simulink model "IEEE34bus_2subsystem"  (R2022b)
settings: Solver=ode4  StartTime=0.0  StopTime=inf  FixedStep=Ts  MaxStep=1e-4  RelTol=1e-4
InitFcn:
  | a=1; % Loading Factor
  | Ts=50e-6;
  | % phase to sequence conversion of RXB matrices
  | c=1*exp(sqrt(-1)*(120*pi/180));
  | T=[1 1 1;1 c*c c;1 c c*c];
  | Tinv=1/3*[1 1 1;1 c c*c;1 c*c c];
  | 
  | % Simulation data for the IEEE 34 Node Test Feeder model
  | mi2km = 1.60934;%  miles to km conversion
  | ft2km = 0.0003048; % feet to km conversion
  | ms2F = 1*1e-6/(2*pi*60);% microsiemens to Farads conversion
  | 
  | %% Configuration 300 - series reactance - ohm/mile
  | R_300 = [1.3368 0.2101 0.2130;0.2101 1.3238 0.2066;0.2130 0.2066 1.3294];
  | X_300 = [1.3343 0.5779 0.5015;0.5779 1.3569 0.4591;0.5015 0.4591 1.3471];
  | % charging susceptance - microsiemens/mile
  | B_300 = [5.3350 -1.5313 -0.9943;-1.5313 5.0979 -0.6212;-0.9943 -0.6212 4.8880];
  | 
  | R_300 = R_300/mi2km;
  | Rseq=Tinv*R_300*T;
  | R1_300=Rseq(2,2);R0_300=Rseq(1,1);
  | 
  | L_300 = (X_300/(2*pi*60))/mi2km;
  | Lseq=Tinv*L_300*T;
  | L1_300=Lseq(2,2);L0_300=Lseq(1,1);
  | 
  | C_300 =(B_300*ms2F)/mi2km;
  | Cseq=Tinv*C_300*T;
  | C1_300=Cseq(2,2);C0_300=Cseq(1,1);
  | 
  | %% Configuration 301 - series reactance - ohm/mile
  | R_301 = [1.9300 0.2327 0.2359;0.2327 1.9157 0.2288;0.2359 0.2288 1.9219];
  | X_301 = [1.4115 0.6442 0.5691;0.6442 1.4281 0.5238;0.5691 0.5238 1.4209];
  | % charging susceptance - microsiemens/mile
  | B_301 = [5.1207 -1.4364 -0.9402;-1.4364 4.9055 -0.5951;-0.9402 -0.5951 4.7154];
  | 
  | R_301 = R_301/mi2km;
  | Rseq=Tinv*R_301*T;
  | R1_301=Rseq(2,2);R0_301=Rseq(1,1);
  | 
  | L_301 = (X_301/(2*pi*60))/mi2km;
  | Lseq=Tinv*L_301*T;
  | L1_301=Lseq(2,2);L0_301=Lseq(1,1);
  | 
  | C_301 =(B_301*ms2F)/mi2km;
  | Cseq=Tinv*C_301*T;
  | C1_301=Cseq(2,2);C0_301=Cseq(1,1);
  | 
  | %% Configuration 302 - series reactance - ohm/mile
  | R_302 = [2.7995 0 0;0 0 0;0 0 0];
  | X_302 = [1.4855 0 0;0 0 0;0 0 0];
  | % charging susceptance - microsiemens/mile
  | B_302 = [4.2251 0 0;0 0 0;0 0 0];
  | 
  | R_302 = R_302/mi2km;
  | Rseq=Tinv*R_302*T;
  | R1_302=Rseq(2,2);R0_302=Rseq(1,1);
  | 
  | L_302 = (X_302/(2*pi*60))/mi2km;
  | Lseq=Tinv*L_302*T;
  | ... (+41 lines)
undefined symbols (not defined in the file): find_system, I, Left, MOV_segment19, MOV_segment9, powergui, Right, type, V, X, xn_g1
libraries: spsSeriesRLCBranchLib x75, spsGroundLib x70, spsThreePhaseVIMeasurementLib x37, spsVoltageMeasurementLib x36, spsThreePhaseSeriesRLCLoadLib x32, spsThreePhasePISectionLineLib x24, spsDCVoltageSourceLib x24, ssn_lib x16, spsSeriesRLCLoadLib x14, spsACCurrentSourceLib x12, spsOnDelayLib x12, spsPiSectionLineLib x8
(part 4 of 8)

== system IEEE34bus_2subsystem/SM_34p/Regulator 3/Single Phase SVR_A/Transformer with Taps ==
  note: Vsec on Pt Ratio base
  note: Isec on CT Ratio base
  N : Inport
  "   " : Terminator
  "    " : Gain  Gain=1/ptRatio
  " 1" : Gain  Gain=-1/ctRatio
  Back-Euler : Constant
  CT1 : spsCurrentMeasurementLib/Current Measurement  PhasorSimulation=off  OutputType=Complex  PSBequivalent=0
  Fcn : Fcn  Expr=1+0.1*u(1)/16
  Ground1 : spsGroundLib/Ground  LConnTagsString=a
  Memory : Memory
  Memory1 : Memory
  Mux1 : Mux  Inputs=2
  PT : spsVoltageMeasurementLib/Voltage Measurement  PhasorSimulation=off  OutputType=Complex  PSBequivalent=0
  SSN Interface Block (1ph) : ssn_lib/SSN Interface Block (1ph)  nb_phase=1  nb_port=2  p1_type=I-type(Left)  p2_type=X-type(Right)  p3_type=V-type(Left)  p4_type=V-type(Left)  p5_type=V-type(Left)  p6_type=V-type(Left)  p7_type=V-type(Left)  p8_type=V-type(Left)  p9_type=V-type(Left)  p10_type=V-type(Left)  p11_type=V-type(Left)  p12_type=V-type(Left)  p13_type=V-type(Left)  p14_type=V-type(Left)  p15_type=V-type(Left)  p16_type=V-type(Left)  I_port_shunt_resistance=1e9
  SSN Interface Block (1ph)2 : ssn_lib/SSN Interface Block (1ph)  nb_phase=1  nb_port=2  p1_type=X-type(Left)  p2_type=I-type(Right)  p3_type=X-type(Left)  p4_type=V-type (Right)  p5_type=V-type(Left)  p6_type=V-type(Left)  p7_type=V-type(Left)  p8_type=V-type(Left)  p9_type=V-type(Left)  p10_type=V-type(Left)  p11_type=V-type(Left)  p12_type=V-type(Left)  p13_type=V-type(Left)  p14_type=V-type(Left)  p15_type=V-type(Left)  p16_type=V-type(Left)  I_port_shunt_resistance=1e9
  SSN OLTC xfo v2 : Subsystem  AncestorBlock=artemis/SSN/SSN OLTC/SSN OLTC xfo v2  mask(Norton-Type External Nodal Subsystem){nnode=2, taggg=ce4x9218xa137594c517a, conntype=2 ports, RLpri=[1e-3 1e-4], Rcore=10000, ensat=off, Lcore=100, Lsat=1, phisat=100, Ts=Ts}
      mask prompts: nnode "Number of Electric nodes"; taggg "Unique Tag Identifier (automatic)"; conntype "Connection type"; RLpri "Primary winding resistance and inductance ([Ohms H])"; Rcore "Core Resistance (Ohms)"; ensat "Enable Saturation"; Lcore "Unsaturated magnetisation inductance (H)"; Lsat "Saturated magnetisation inductance (H)"; phisat "Flux saturation threshold (Weber)"; Ts "Sample Time (s)"
      mask help:
      | Continuously-variable On-Load Tapped Transformer (OLTC) (SSN Custom model)
      |
      | This block implements a 2 winding OLTC saturable transformer in SSN.
      | The model has a variable secondary inductance and resistance as well as turn-ratio.
      | The secondary winding is on the side marked with 'TAP'
      |
      | Mask parameters:
      |    Unique Tag Identifier: unique tag required by SSN to recknonize SSN external models
      |    Primary winding resistance and inductance ([Ohms H])
      |    Core Resistance (Ohms)
      |    Unsaturated magnetisation inductance (H): unsaturated core magnetization inductance
      |    Saturated magnetisation inductance (H): local inductance of the core in the saturated region
      |    Flux saturation threshold (Weber): flux saturation point
      |
      | Signal parameters:
      |
      | Signal inputs:
      |    1st sig: secondary winding resistance (Ohms)
      |    2nd sig: secondary winding inductance (H)
      |    3rd sig: transformer turn ratio k (V_secondary_tapped=k*V_primary)
      |    4th sig:  when set to 1, uses the Backward Euler method for solver. This can be used dynamically during simulation for example to damp numerical oscillations after switching events or after tap changes.
      |
      | Signals ouputs:
      |    1st signal: primary input current (A)
      |    2nd signal: secondary winding current (A)
      |    3rd signal: transformer flux (Wb)
      |
      | Saturation characteristic:
      |          flux
      |             ^              2
      |             |      1       *   <--- slope between point1 and point2 is Lsaturated
      |  phisat  |-----*  <---  this is the knee of flux=f(imag)
      |             |
      |             |
      |             |  <-----slope between origin and point1 is Lunsaturated
      |             *-------------------> imag
      mask init:
      | bloc=gcb;
      | taggg=get_param(bloc,'taggg');
      | conntyp=get_param(bloc,'conntype');
      | set_param([bloc '/FromV'],'GotoTag',['ssn_ext_sys_from_V_' taggg]);
      | set_param([bloc '/GotoHist'],'GotoTag',['ssn_ext_sys_goto_Hist_' taggg]);
      | set_param([bloc '/GotoY'],'GotoTag',['ssn_ext_sys_goto_Y_' taggg]);
      | 
      | R1=RLpri(1);
      | L1=RLpri(2);
      | 
      | if isequal(get_param(bloc,'ensat'),'off')
      |     phisat=1e20;
      | end
      | 
      | if isequal(conntyp,'4 ports')
      |     vin_sel=[1 2 3 4];
      |     Vinzeros=0;
      |     hist_sel=[1 2 3 4];
      |     a1=0;a2=0;a3=100;a4=100; b1=[7,34,40,33,31,33,40,33,31,33,40,33,31,33,40,34,7];b2=[30,30,34,42,40,37,45,52,50,47,54,62,59,57,65,70,70];b3=[93,67,60,67,70,67,60,67,70,67,60,67,70,67,60,67,93];b4=[30,30,34,42,40,37,45,52,50,47,54,62,60,57,65,70,70];
      |     c1=[20,20]*0;c2=[20,30]*0;c3=[27,14]*0;c4=[20,20]*0;c5=[24,17]*0;c6=[16,16]*0;c7=[22,19]*0;c8=[13,13]*0;c9=[80,80]*0;c10=[20,30]*0;c11=[88,74]*0;c12=[20,20]*0;c13=[85,77]*0;c14=[16,16]*0;c15=[81,79]*0;c16=[13,13]*0;
      |     %d1=[85,80];d2=[60,60];d3=[83,83];d4=[50,60];d5=[90,88,86];d6=[50,60,50];d7=[89,87];d8=[54,54];d9=[92,95,96,96,95,92,92];d10=[53,53,55,58,60,60,50];
      | 
      | 
      | elseif isequal(conntyp,'3 ports (primary grounded)')
      |     vin_sel=[1 2 5 3];
      |     Vinzeros=[0 0];
      |     hist_sel=[1 2 4];
      |   
      |      a1=0;a2=0;a3=100;a4=100; b1=[20,34,40,33,31,33,40,33,31,33,40,33,31,33,40,34,7];b2=[30,30,34,42,40,37,45,52,50,47,54,62,59,57,65,70,70];b3=[93,67,60,67,70,67,60,67,70,67,60,67,70,67,60,67,93];b4=[30,30,34,42,40,37,45,52,50,47,54,62,60,57,65,70,70];
      |     c1=[20,20];c2=[20,30];c3=[27,14];c4=[20,20];c5=[24,17];c6=[16,16];c7=[22,19];c8=[13,13];c9=[80,80]*0;c10=[20,30]*0;c11=[88,74]*0;c12=[20,20]*0;c13=[85,77]*0;c14=[16,16]*0;c15=[81,79]*0;c16=[13,13]*0;
      |     %d1=[85,80];d2=[60,60];d3=[83,83];d4=[50,60];d5=[90,88,86];d6=[50,60,50];d7=[89,87];d8=[54,54];d9=[92,95,96,96,95,92,92];d10=[53,53,55,58,60,60,50];
      | elseif isequal(conntyp,'3 ports (tapped secondary grounded)')
      |     vin_sel=[1 2 3 5];
      |     Vinzeros=[0 0];
      |     hist_sel=[1 2 3];
      |  
      |    a1=0;a2=0;a3=100;a4=100; b1=[20,34,40,33,31,33,40,33,31,33,40,33,31,33,40,34,7];b2=[30,30,34,42,40,37,45,52,50,47,54,62,59,57,65,70,70];b3=[80,67,60,67,70,67,60,67,70,67,60,67,70,67,60,67,93];b4=[30,30,34,42,40,37,45,52,50,47,54,62,60,57,65,70,70];
      |     c1=[20,20]*0;c2=[20,30]*0;c3=[27,14]*0;c4=[20,20]*0;c5=[24,17]*0;c6=[16,16]*0;c7=[22,19]*0;c8=[13,13]*0;c9=[80,80];c10=[20,30];c11=[88,74];c12=[20,20];c13=[85,77];c14=[16,16];c15=[81,79];c16=[13,13];
      |     %d1=[85,80];d2=[60,60];d3=[83,83];d4=[50,60];d5=[90,88,86];d6=[50,60,50];d7=[89,87];d8=[54,54];d9=[92,95,96,96,95,92,92];d10=[53,53,55,58,60,60,50];
      | elseif isequal(conntyp,'2 ports')
      |     vin_sel=[1 2 5 5];
      |     Vinzeros=[0 0 0];
      |     hist_sel=[1 2];
      |         a1=0;a2=0;a3=100;a4=100; b1=[20,34,40,33,31,33,40,33,31,33,40,33,31,33,40,34,7];b2=[30,30,34,42,40,37,45,52,50,47,54,62,59,57,65,70,70];b3=[80,67,60,67,70,67,60,67,70,67,60,67,70,67,60,67,93];b4=[30,30,34,42,40,37,45,52,50,47,54,62,60,57,65,70,70];
      |     c1=[20,20];c2=[20,30];c3=[27,14];c4=[20,20];c5=[24,17];c6=[16,16];c7=[22,19];c8=[13,13];c9=[80,80];c10=[20,30];c11=[88,74];c12=[20,20];c13=[85,77];c14=[16,16];c15=[81,79];c16=[13,13];
      |     %d1=[85,80];d2=[60,60];d3=[83,83];d4=[50,60];d5=[90,88,86];d6=[50,60,50];d7=[89,87];d8=[54,54];d9=[92,95,96,96,95,92,92];d10=[53,53,55,58,60,60,50];
      | else
      | 
      | end
      | 
      | ori=get_param(bloc,'Orientation');
      | 
      | if isequal(ori,'right')
      |     d1=[73,67];d2=[56,56];d3=[70,70];d4=[45,56];d5=[80,77,75];d6=[45,56,45];d7=[79,76];d8=[50,50];d9=[82,84,86,84,82,82];d10=[50,50,54,56,56,45];
      | else
      |     d1=[73,71,69,71,73,73];d2=[50,50,52,56,56,45];d3=[80,77,75];d4=[45,56,45];d5=[76,79];d6=[50,50];d7=[88,82];d8=[56,56];d9=[85,85];d10=[45,56];
      | end
      settings: LibrarySourceBlock=artemis/SSN/SSN OLTC/SSN OLTC xfo v2
      settings: CopyFcn=|
      | str=tempname;
      | str=strrep(str(end-20:end),'_','x');
      | set_param(gcb,'taggg',str);
      | set_param(gcb,'LinkStatus','inactive');
      mask Help: eval('open SSN_OLTC.pdf;');
      mask TypeOptions conntype: 4 ports | 3 ports (primary grounded) | 3 ports (tapped secondary grounded) | 2 ports
      mask Callback conntype:
      | bloc=gcb;
      | conntyp=get_param(bloc,'conntype');
      | nn=fts6_xfo_port_cb(bloc,conntyp);
      | set_param(bloc,'nnode',nn);
      mask Display:
      | plot(a1,a2,a3,a4,b1,b2,b3,b4,c1,c2,c3,c4,c5,c6,c7,c8,c9,c10,c11,c12,c13,c14,c15,c16);
      | color('blue');
      | plot(d1,d2,d3,d4,d5,d6,d7,d8,d9,d10);
  Transfo R2-L2-turnratio : Constant  Value=[0.0001 0.00001 1]
  x : Product  RndMeth=Zero
  L : PMIOPort  Tag=PMCPort  Side=Right
  S : PMIOPort  Port=2  Side=Left
  Isec : Outport
  Vsec : Outport  Port=2
  wires:
  Fcn/1 -> x/1
  Mux1/1 -> SSN OLTC xfo v2/1(params)
  x/1 -> Mux1/1
  Transfo R2-L2-turnratio/1 -> x/2
  Back-Euler/1 -> Mux1/2
  SSN OLTC xfo v2/1(meas) -> "   "/1  "transfo flux (Weber)"
  N/1 -> Fcn/1
  "    "/1 -> Memory1/1
  PT/1 -> "    "/1
  CT1/1 -> " 1"/1
  " 1"/1 -> Memory/1
  Memory1/1 -> Vsec/1
  Memory/1 -> Isec/1
  connections:
  CT1/RConn1 -- SSN Interface Block (1ph)2/RConn1 -- PT/LConn1
  SSN OLTC xfo v2/LConn1 -- SSN Interface Block (1ph)/RConn1
  SSN OLTC xfo v2/RConn1 -- SSN Interface Block (1ph)2/LConn1
  S/RConn1 -- SSN Interface Block (1ph)/LConn1
  PT/LConn2 -- Ground1/LConn1
  CT1/LConn1 -- L/RConn1

== system IEEE34bus_2subsystem/SM_34p/Regulator 3/Single Phase SVR_A/Voltage Regulator Control ==
  Vm : Inport
  Constant : Constant  Value=RegulatorOn
  Tap Changer Control : Subsystem  mask(Tap Changer Control){MinMaxTap=TapMinMax, InitialPosition=InitialTap, MecDelay=TapSelectionTime}
      mask prompts: MinMaxTap "Minimum and maximum tap number [ Min  Max ] :"; InitialPosition "Initial tap position"; MecDelay "Mechanical delay time"
      mask init:
      | if MecDelay<=0,
      | 	MecDelay=1/60;
      | end
  Voltage regulator : Subsystem  mask{Vref=RegulatorVref*120, DeadBand=RegulatorDeadBand*120, TimeDelay=RegulatorDelay}
      mask prompts: Vref "Vref (on 120v base)"; DeadBand "Deadband (on 120v base)"; TimeDelay "Time delay (s)"
  N : Outport
  Tap : Outport  Port=2
  wires:
  Voltage regulator/2(Down) -> Tap Changer Control/2("Down ")
  Tap Changer Control/1(TapNo) -> Tap/1, N/1  "Tap"
  Voltage regulator/1(Up) -> Tap Changer Control/1("Up ")
  Tap Changer Control/2(Ready) -> Voltage regulator/2(Ready)
  Constant/1 -> Voltage regulator/3(RegOn)
  Vm/1 -> Voltage regulator/1(Vmes (pu))

== system IEEE34bus_2subsystem/SM_34p/Regulator 3/Single Phase SVR_B/Line Drop Compensator ==
  note: Vm=Vsec-Isec(Rc+jXc)
  Isec : Inport
  Vsec : Inport  Port=2
  "        " : spsLinearTransformerLib/Linear Transformer  UNITS=SI  NominalPower=[pNom fNom]  winding1=[vNom/ptRatio 1e-7 1e-8]  winding2=[vNom/ptRatio 1e-7 1e-8]  ThreeWindings=off  winding3=[3.15e+005 0.7938 0.084225]  RmLm=[1e5 1e5]  Measurements=None  DataType=on
  "CTS  " : spsControlledCurrentSourceLib/Controlled Current Source  Initialize=on  Source_Type=AC  Amplitude=0  Phase=0  Frequency=0  Measurements=None
  "PTS  " : spsControlledVoltageSourceLib/Controlled Voltage Source  Initialize=on  Source_Type=AC  Amplitude=0  Phase=0  Frequency=0  Measurements=None
  RMS : spsRMSLib/RMS  TrueRMS=on  Freq=60  RMSInit=120  Ts=0
  Raux : spsSeriesRLCBranchLib/Series RLC Branch  LConnTagsString=__new0  RConnTagsString=__new0  BranchType=R  Resistance=1e3  Inductance=1.6 / (120*pi)  SetiL0=off  InitialCurrent=0  Capacitance=1e-6  Setx0=off  InitialVoltage=0  Measurements=None
  Rc+jXc : spsSeriesRLCBranchLib/Series RLC Branch  LConnTagsString=__new0  RConnTagsString=__new0  BranchType=RL  Resistance=Rc  Inductance=Xc / (2*pi*fNom)  SetiL0=off  InitialCurrent=0  Capacitance=1e-6  Setx0=off  InitialVoltage=0  Measurements=None
  VRelay : spsVoltageMeasurementLib/Voltage Measurement  PhasorSimulation=off  OutputType=Complex  PSBequivalent=0
  Vm : Outport
  wires:
  RMS/1 -> Vm/1
  VRelay/1 -> RMS/1
  Isec/1 -> "CTS  "/1
  Vsec/1 -> "PTS  "/1
  connections:
  "PTS  "/RConn1 -- "        "/RConn1
  "        "/RConn2 -- VRelay/LConn1
  Raux/LConn1 -- Rc+jXc/LConn1 -- "        "/LConn1 -- "CTS  "/RConn1
  Rc+jXc/RConn1 -- Raux/RConn1 -- "CTS  "/LConn1 -- "        "/LConn2
  VRelay/LConn2 -- "PTS  "/LConn1

== system IEEE34bus_2subsystem/SM_34p/Regulator 3/Single Phase SVR_B/Transformer with Taps ==
  note: Isec on CT Ratio base
  note: Vsec on Pt Ratio base
  N : Inport
  "   " : Terminator
  "    " : Gain  Gain=1/ptRatio
  " 1" : Gain  Gain=-1/ctRatio
  Back-Euler : Constant
  CT1 : spsCurrentMeasurementLib/Current Measurement  PhasorSimulation=off  OutputType=Complex  PSBequivalent=0
  Fcn : Fcn  Expr=1+0.1*u(1)/16
  Ground1 : spsGroundLib/Ground  LConnTagsString=a
  Memory : Memory
  Memory1 : Memory
  Mux1 : Mux  Inputs=2
  PT : spsVoltageMeasurementLib/Voltage Measurement  PhasorSimulation=off  OutputType=Complex  PSBequivalent=0
  SSN Interface Block (1ph) : ssn_lib/SSN Interface Block (1ph)  nb_phase=1  nb_port=2  p1_type=I-type(Left)  p2_type=X-type(Right)  p3_type=V-type(Left)  p4_type=V-type(Left)  p5_type=V-type(Left)  p6_type=V-type(Left)  p7_type=V-type(Left)  p8_type=V-type(Left)  p9_type=V-type(Left)  p10_type=V-type(Left)  p11_type=V-type(Left)  p12_type=V-type(Left)  p13_type=V-type(Left)  p14_type=V-type(Left)  p15_type=V-type(Left)  p16_type=V-type(Left)  I_port_shunt_resistance=1e9
  SSN Interface Block (1ph)2 : ssn_lib/SSN Interface Block (1ph)  nb_phase=1  nb_port=2  p1_type=X-type(Left)  p2_type=I-type(Right)  p3_type=X-type(Left)  p4_type=V-type (Right)  p5_type=V-type(Left)  p6_type=V-type(Left)  p7_type=V-type(Left)  p8_type=V-type(Left)  p9_type=V-type(Left)  p10_type=V-type(Left)  p11_type=V-type(Left)  p12_type=V-type(Left)  p13_type=V-type(Left)  p14_type=V-type(Left)  p15_type=V-type(Left)  p16_type=V-type(Left)  I_port_shunt_resistance=1e9
  SSN OLTC xfo v2 : Subsystem  AncestorBlock=artemis/SSN/SSN OLTC/SSN OLTC xfo v2  mask(Norton-Type External Nodal Subsystem){nnode=2, taggg=687x9d5fx6fb80ff9f5a3, conntype=2 ports, RLpri=[1e-3 1e-4], Rcore=10000, ensat=off, Lcore=100, Lsat=1, phisat=100, Ts=Ts}
      mask prompts: nnode "Number of Electric nodes"; taggg "Unique Tag Identifier (automatic)"; conntype "Connection type"; RLpri "Primary winding resistance and inductance ([Ohms H])"; Rcore "Core Resistance (Ohms)"; ensat "Enable Saturation"; Lcore "Unsaturated magnetisation inductance (H)"; Lsat "Saturated magnetisation inductance (H)"; phisat "Flux saturation threshold (Weber)"; Ts "Sample Time (s)"
      mask help:
      | Continuously-variable On-Load Tapped Transformer (OLTC) (SSN Custom model)
      |
      | This block implements a 2 winding OLTC saturable transformer in SSN.
      | The model has a variable secondary inductance and resistance as well as turn-ratio.
      | The secondary winding is on the side marked with 'TAP'
      |
      | Mask parameters:
      |    Unique Tag Identifier: unique tag required by SSN to recknonize SSN external models
      |    Primary winding resistance and inductance ([Ohms H])
      |    Core Resistance (Ohms)
      |    Unsaturated magnetisation inductance (H): unsaturated core magnetization inductance
      |    Saturated magnetisation inductance (H): local inductance of the core in the saturated region
      |    Flux saturation threshold (Weber): flux saturation point
      |
      | Signal parameters:
      |
      | Signal inputs:
      |    1st sig: secondary winding resistance (Ohms)
      |    2nd sig: secondary winding inductance (H)
      |    3rd sig: transformer turn ratio k (V_secondary_tapped=k*V_primary)
      |    4th sig:  when set to 1, uses the Backward Euler method for solver. This can be used dynamically during simulation for example to damp numerical oscillations after switching events or after tap changes.
      |
      | Signals ouputs:
      |    1st signal: primary input current (A)
      |    2nd signal: secondary winding current (A)
      |    3rd signal: transformer flux (Wb)
      |
      | Saturation characteristic:
      |          flux
      |             ^              2
      |             |      1       *   <--- slope between point1 and point2 is Lsaturated
      |  phisat  |-----*  <---  this is the knee of flux=f(imag)
      |             |
      |             |
      |             |  <-----slope between origin and point1 is Lunsaturated
      |             *-------------------> imag
      mask init: same as IEEE34bus_2subsystem/SM_34p/Regulator 3/Single Phase SVR_A/Transformer with Taps/SSN OLTC xfo v2
      settings: LibrarySourceBlock=artemis/SSN/SSN OLTC/SSN OLTC xfo v2
      settings: CopyFcn=|
      | str=tempname;
      | str=strrep(str(end-20:end),'_','x');
      | set_param(gcb,'taggg',str);
      | set_param(gcb,'LinkStatus','inactive');
      mask Help: eval('open SSN_OLTC.pdf;');
      mask TypeOptions conntype: 4 ports | 3 ports (primary grounded) | 3 ports (tapped secondary grounded) | 2 ports
      mask Callback conntype:
      | bloc=gcb;
      | conntyp=get_param(bloc,'conntype');
      | nn=fts6_xfo_port_cb(bloc,conntyp);
      | set_param(bloc,'nnode',nn);
      mask Display:
      | plot(a1,a2,a3,a4,b1,b2,b3,b4,c1,c2,c3,c4,c5,c6,c7,c8,c9,c10,c11,c12,c13,c14,c15,c16);
      | color('blue');
      | plot(d1,d2,d3,d4,d5,d6,d7,d8,d9,d10);
  Transfo R2-L2-turnratio : Constant  Value=[0.0001 0.00001 1]
  x : Product  RndMeth=Zero
  L : PMIOPort  Tag=PMCPort  Side=Right
  S : PMIOPort  Port=2  Side=Left
  Isec : Outport
  Vsec : Outport  Port=2
  wires:
  Memory/1 -> Isec/1
  Memory1/1 -> Vsec/1
  " 1"/1 -> Memory/1
  CT1/1 -> " 1"/1
  PT/1 -> "    "/1
  "    "/1 -> Memory1/1
  N/1 -> Fcn/1
  SSN OLTC xfo v2/1(meas) -> "   "/1  "transfo flux (Weber)"
  Back-Euler/1 -> Mux1/2
  Transfo R2-L2-turnratio/1 -> x/2
  x/1 -> Mux1/1
  Mux1/1 -> SSN OLTC xfo v2/1(params)
  Fcn/1 -> x/1
  connections:
  CT1/LConn1 -- L/RConn1
  PT/LConn2 -- Ground1/LConn1
  S/RConn1 -- SSN Interface Block (1ph)/LConn1
  SSN OLTC xfo v2/RConn1 -- SSN Interface Block (1ph)2/LConn1
  SSN OLTC xfo v2/LConn1 -- SSN Interface Block (1ph)/RConn1
  PT/LConn1 -- SSN Interface Block (1ph)2/RConn1 -- CT1/RConn1

== system IEEE34bus_2subsystem/SM_34p/Regulator 3/Single Phase SVR_B/Voltage Regulator Control ==
  Vm : Inport
  Constant : Constant  Value=RegulatorOn
  Tap Changer Control : Subsystem  mask(Tap Changer Control){MinMaxTap=TapMinMax, InitialPosition=InitialTap, MecDelay=TapSelectionTime}
      mask prompts: MinMaxTap "Minimum and maximum tap number [ Min  Max ] :"; InitialPosition "Initial tap position"; MecDelay "Mechanical delay time"
      mask init:
      | if MecDelay<=0,
      | 	MecDelay=1/60;
      | end
  Voltage regulator : Subsystem  mask{Vref=RegulatorVref*120, DeadBand=RegulatorDeadBand*120, TimeDelay=RegulatorDelay}
      mask prompts: Vref "Vref (on 120v base)"; DeadBand "Deadband (on 120v base)"; TimeDelay "Time delay (s)"
  N : Outport
  Tap : Outport  Port=2
  wires:
  Vm/1 -> Voltage regulator/1(Vmes (pu))
  Constant/1 -> Voltage regulator/3(RegOn)
  Tap Changer Control/2(Ready) -> Voltage regulator/2(Ready)
  Voltage regulator/1(Up) -> Tap Changer Control/1("Up ")
  Tap Changer Control/1(TapNo) -> N/1, Tap/1  "Tap"
  Voltage regulator/2(Down) -> Tap Changer Control/2("Down ")

== system IEEE34bus_2subsystem/SM_34p/Regulator 3/Single Phase SVR_C/Line Drop Compensator ==
  note: Vm=Vsec-Isec(Rc+jXc)
  Isec : Inport
  Vsec : Inport  Port=2
  "        " : spsLinearTransformerLib/Linear Transformer  UNITS=SI  NominalPower=[pNom fNom]  winding1=[vNom/ptRatio 1e-7 1e-8]  winding2=[vNom/ptRatio 1e-7 1e-8]  ThreeWindings=off  winding3=[3.15e+005 0.7938 0.084225]  RmLm=[1e5 1e5]  Measurements=None  DataType=on
  "CTS  " : spsControlledCurrentSourceLib/Controlled Current Source  Initialize=on  Source_Type=AC  Amplitude=0  Phase=0  Frequency=0  Measurements=None
  "PTS  " : spsControlledVoltageSourceLib/Controlled Voltage Source  Initialize=on  Source_Type=AC  Amplitude=0  Phase=0  Frequency=0  Measurements=None
  RMS : spsRMSLib/RMS  TrueRMS=on  Freq=60  RMSInit=120  Ts=0
  Raux : spsSeriesRLCBranchLib/Series RLC Branch  LConnTagsString=__new0  RConnTagsString=__new0  BranchType=R  Resistance=1e3  Inductance=1.6 / (120*pi)  SetiL0=off  InitialCurrent=0  Capacitance=1e-6  Setx0=off  InitialVoltage=0  Measurements=None
  Rc+jXc : spsSeriesRLCBranchLib/Series RLC Branch  LConnTagsString=__new0  RConnTagsString=__new0  BranchType=RL  Resistance=Rc  Inductance=Xc / (2*pi*fNom)  SetiL0=off  InitialCurrent=0  Capacitance=1e-6  Setx0=off  InitialVoltage=0  Measurements=None
  VRelay : spsVoltageMeasurementLib/Voltage Measurement  PhasorSimulation=off  OutputType=Complex  PSBequivalent=0
  Vm : Outport
  wires:
  Vsec/1 -> "PTS  "/1
  Isec/1 -> "CTS  "/1
  VRelay/1 -> RMS/1
  RMS/1 -> Vm/1
  connections:
  VRelay/LConn2 -- "PTS  "/LConn1
  "        "/LConn2 -- "CTS  "/LConn1 -- Raux/RConn1 -- Rc+jXc/RConn1
  "CTS  "/RConn1 -- "        "/LConn1 -- Rc+jXc/LConn1 -- Raux/LConn1
  "        "/RConn2 -- VRelay/LConn1
  "PTS  "/RConn1 -- "        "/RConn1

== system IEEE34bus_2subsystem/SM_34p/Regulator 3/Single Phase SVR_C/Transformer with Taps ==
  note: Vsec on Pt Ratio base
  note: Isec on CT Ratio base
  N : Inport
  "   " : Terminator
  "    " : Gain  Gain=1/ptRatio
  " 1" : Gain  Gain=-1/ctRatio
  Back-Euler : Constant
  CT1 : spsCurrentMeasurementLib/Current Measurement  PhasorSimulation=off  OutputType=Complex  PSBequivalent=0
  Fcn : Fcn  Expr=1+0.1*u(1)/16
  Ground1 : spsGroundLib/Ground  LConnTagsString=a
  Memory : Memory
  Memory1 : Memory
  Mux1 : Mux  Inputs=2
  PT : spsVoltageMeasurementLib/Voltage Measurement  PhasorSimulation=off  OutputType=Complex  PSBequivalent=0
  SSN Interface Block (1ph) : ssn_lib/SSN Interface Block (1ph)  nb_phase=1  nb_port=2  p1_type=I-type(Left)  p2_type=X-type(Right)  p3_type=V-type(Left)  p4_type=V-type(Left)  p5_type=V-type(Left)  p6_type=V-type(Left)  p7_type=V-type(Left)  p8_type=V-type(Left)  p9_type=V-type(Left)  p10_type=V-type(Left)  p11_type=V-type(Left)  p12_type=V-type(Left)  p13_type=V-type(Left)  p14_type=V-type(Left)  p15_type=V-type(Left)  p16_type=V-type(Left)  I_port_shunt_resistance=1e9
  SSN Interface Block (1ph)2 : ssn_lib/SSN Interface Block (1ph)  nb_phase=1  nb_port=2  p1_type=X-type(Left)  p2_type=I-type(Right)  p3_type=X-type(Left)  p4_type=V-type (Right)  p5_type=V-type(Left)  p6_type=V-type(Left)  p7_type=V-type(Left)  p8_type=V-type(Left)  p9_type=V-type(Left)  p10_type=V-type(Left)  p11_type=V-type(Left)  p12_type=V-type(Left)  p13_type=V-type(Left)  p14_type=V-type(Left)  p15_type=V-type(Left)  p16_type=V-type(Left)  I_port_shunt_resistance=1e9
  SSN OLTC xfo v2 : Subsystem  AncestorBlock=artemis/SSN/SSN OLTC/SSN OLTC xfo v2  mask(Norton-Type External Nodal Subsystem){nnode=2, taggg=e41xb614x261f7399655c, conntype=2 ports, RLpri=[1e-3 1e-4], Rcore=10000, ensat=off, Lcore=100, Lsat=1, phisat=100, Ts=Ts}
      mask prompts: nnode "Number of Electric nodes"; taggg "Unique Tag Identifier (automatic)"; conntype "Connection type"; RLpri "Primary winding resistance and inductance ([Ohms H])"; Rcore "Core Resistance (Ohms)"; ensat "Enable Saturation"; Lcore "Unsaturated magnetisation inductance (H)"; Lsat "Saturated magnetisation inductance (H)"; phisat "Flux saturation threshold (Weber)"; Ts "Sample Time (s)"
      mask help:
      | Continuously-variable On-Load Tapped Transformer (OLTC) (SSN Custom model)
      |
      | This block implements a 2 winding OLTC saturable transformer in SSN.
      | The model has a variable secondary inductance and resistance as well as turn-ratio.
      | The secondary winding is on the side marked with 'TAP'
      |
      | Mask parameters:
      |    Unique Tag Identifier: unique tag required by SSN to recknonize SSN external models
      |    Primary winding resistance and inductance ([Ohms H])
      |    Core Resistance (Ohms)
      |    Unsaturated magnetisation inductance (H): unsaturated core magnetization inductance
      |    Saturated magnetisation inductance (H): local inductance of the core in the saturated region
      |    Flux saturation threshold (Weber): flux saturation point
      |
      | Signal parameters:
      |
      | Signal inputs:
      |    1st sig: secondary winding resistance (Ohms)
      |    2nd sig: secondary winding inductance (H)
      |    3rd sig: transformer turn ratio k (V_secondary_tapped=k*V_primary)
      |    4th sig:  when set to 1, uses the Backward Euler method for solver. This can be used dynamically during simulation for example to damp numerical oscillations after switching events or after tap changes.
      |
      | Signals ouputs:
      |    1st signal: primary input current (A)
      |    2nd signal: secondary winding current (A)
      |    3rd signal: transformer flux (Wb)
      |
      | Saturation characteristic:
      |          flux
      |             ^              2
      |             |      1       *   <--- slope between point1 and point2 is Lsaturated
      |  phisat  |-----*  <---  this is the knee of flux=f(imag)
      |             |
      |             |
      |             |  <-----slope between origin and point1 is Lunsaturated
      |             *-------------------> imag
      mask init: same as IEEE34bus_2subsystem/SM_34p/Regulator 3/Single Phase SVR_A/Transformer with Taps/SSN OLTC xfo v2
      settings: LibrarySourceBlock=artemis/SSN/SSN OLTC/SSN OLTC xfo v2
      settings: CopyFcn=|
      | str=tempname;
      | str=strrep(str(end-20:end),'_','x');
      | set_param(gcb,'taggg',str);
      | set_param(gcb,'LinkStatus','inactive');
      mask Help: eval('open SSN_OLTC.pdf;');
      mask TypeOptions conntype: 4 ports | 3 ports (primary grounded) | 3 ports (tapped secondary grounded) | 2 ports
      mask Callback conntype:
      | bloc=gcb;
      | conntyp=get_param(bloc,'conntype');
      | nn=fts6_xfo_port_cb(bloc,conntyp);
      | set_param(bloc,'nnode',nn);
      mask Display:
      | plot(a1,a2,a3,a4,b1,b2,b3,b4,c1,c2,c3,c4,c5,c6,c7,c8,c9,c10,c11,c12,c13,c14,c15,c16);
      | color('blue');
      | plot(d1,d2,d3,d4,d5,d6,d7,d8,d9,d10);
  Transfo R2-L2-turnratio : Constant  Value=[0.0001 0.00001 1]
  x : Product  RndMeth=Zero
  L : PMIOPort  Tag=PMCPort  Side=Right
  S : PMIOPort  Port=2  Side=Left
  Isec : Outport
  Vsec : Outport  Port=2
  wires:
  Fcn/1 -> x/1
  Mux1/1 -> SSN OLTC xfo v2/1(params)
  x/1 -> Mux1/1
  Transfo R2-L2-turnratio/1 -> x/2
  Back-Euler/1 -> Mux1/2
  SSN OLTC xfo v2/1(meas) -> "   "/1  "transfo flux (Weber)"
  N/1 -> Fcn/1
  "    "/1 -> Memory1/1
  PT/1 -> "    "/1
  CT1/1 -> " 1"/1
  " 1"/1 -> Memory/1
  Memory1/1 -> Vsec/1
  Memory/1 -> Isec/1
  connections:
  CT1/RConn1 -- SSN Interface Block (1ph)2/RConn1 -- PT/LConn1
  SSN OLTC xfo v2/LConn1 -- SSN Interface Block (1ph)/RConn1
  SSN OLTC xfo v2/RConn1 -- SSN Interface Block (1ph)2/LConn1
  S/RConn1 -- SSN Interface Block (1ph)/LConn1
  PT/LConn2 -- Ground1/LConn1
  CT1/LConn1 -- L/RConn1

== system IEEE34bus_2subsystem/SM_34p/Regulator 3/Single Phase SVR_C/Voltage Regulator Control ==
  Vm : Inport
  Constant : Constant  Value=RegulatorOn
  Tap Changer Control : Subsystem  mask(Tap Changer Control){MinMaxTap=TapMinMax, InitialPosition=InitialTap, MecDelay=TapSelectionTime}
      mask prompts: MinMaxTap "Minimum and maximum tap number [ Min  Max ] :"; InitialPosition "Initial tap position"; MecDelay "Mechanical delay time"
      mask init:
      | if MecDelay<=0,
      | 	MecDelay=1/60;
      | end
  Voltage regulator : Subsystem  mask{Vref=RegulatorVref*120, DeadBand=RegulatorDeadBand*120, TimeDelay=RegulatorDelay}
      mask prompts: Vref "Vref (on 120v base)"; DeadBand "Deadband (on 120v base)"; TimeDelay "Time delay (s)"
  N : Outport
  Tap : Outport  Port=2
  wires:
  Voltage regulator/2(Down) -> Tap Changer Control/2("Down ")
  Tap Changer Control/1(TapNo) -> Tap/1, N/1  "Tap"
  Voltage regulator/1(Up) -> Tap Changer Control/1("Up ")
  Tap Changer Control/2(Ready) -> Voltage regulator/2(Ready)
  Constant/1 -> Voltage regulator/3(RegOn)
  Vm/1 -> Voltage regulator/1(Vmes (pu))

== system IEEE34bus_2subsystem/SM_34p/Regulator 4/Single Phase SVR_A/Line Drop Compensator ==
  note: Vm=Vsec-Isec(Rc+jXc)
  Isec : Inport
  Vsec : Inport  Port=2
  "        " : spsLinearTransformerLib/Linear Transformer  UNITS=SI  NominalPower=[pNom fNom]  winding1=[vNom/ptRatio 1e-7 1e-8]  winding2=[vNom/ptRatio 1e-7 1e-8]  ThreeWindings=off  winding3=[3.15e+005 0.7938 0.084225]  RmLm=[1e5 1e5]  Measurements=None  DataType=on
  "CTS  " : spsControlledCurrentSourceLib/Controlled Current Source  Initialize=on  Source_Type=AC  Amplitude=0  Phase=0  Frequency=0  Measurements=None
  "PTS  " : spsControlledVoltageSourceLib/Controlled Voltage Source  Initialize=on  Source_Type=AC  Amplitude=0  Phase=0  Frequency=0  Measurements=None
  RMS : spsRMSLib/RMS  TrueRMS=on  Freq=60  RMSInit=120  Ts=0
  Raux : spsSeriesRLCBranchLib/Series RLC Branch  LConnTagsString=__new0  RConnTagsString=__new0  BranchType=R  Resistance=1e3  Inductance=1.6 / (120*pi)  SetiL0=off  InitialCurrent=0  Capacitance=1e-6  Setx0=off  InitialVoltage=0  Measurements=None
  Rc+jXc : spsSeriesRLCBranchLib/Series RLC Branch  LConnTagsString=__new0  RConnTagsString=__new0  BranchType=RL  Resistance=Rc  Inductance=Xc / (2*pi*fNom)  SetiL0=off  InitialCurrent=0  Capacitance=1e-6  Setx0=off  InitialVoltage=0  Measurements=None
  VRelay : spsVoltageMeasurementLib/Voltage Measurement  PhasorSimulation=off  OutputType=Complex  PSBequivalent=0
  Vm : Outport
  wires:
  RMS/1 -> Vm/1
  VRelay/1 -> RMS/1
  Isec/1 -> "CTS  "/1
  Vsec/1 -> "PTS  "/1
  connections:
  "PTS  "/RConn1 -- "        "/RConn1
  "        "/RConn2 -- VRelay/LConn1
  Raux/LConn1 -- Rc+jXc/LConn1 -- "        "/LConn1 -- "CTS  "/RConn1
  Rc+jXc/RConn1 -- Raux/RConn1 -- "CTS  "/LConn1 -- "        "/LConn2
  VRelay/LConn2 -- "PTS  "/LConn1

== system IEEE34bus_2subsystem/SM_34p/Regulator 4/Single Phase SVR_A/Transformer with Taps ==
  note: Isec on CT Ratio base
  note: Vsec on Pt Ratio base
  N : Inport
  "   " : Terminator
  "    " : Gain  Gain=1/ptRatio
  " 1" : Gain  Gain=-1/ctRatio
  Back-Euler : Constant
  CT1 : spsCurrentMeasurementLib/Current Measurement  PhasorSimulation=off  OutputType=Complex  PSBequivalent=0
  Fcn : Fcn  Expr=1+0.1*u(1)/16
  Ground1 : spsGroundLib/Ground  LConnTagsString=a
  Memory : Memory
  Memory1 : Memory
  Mux1 : Mux  Inputs=2
  PT : spsVoltageMeasurementLib/Voltage Measurement  PhasorSimulation=off  OutputType=Complex  PSBequivalent=0
  SSN Interface Block (1ph) : ssn_lib/SSN Interface Block (1ph)  nb_phase=1  nb_port=2  p1_type=I-type(Left)  p2_type=X-type(Right)  p3_type=V-type(Left)  p4_type=V-type(Left)  p5_type=V-type(Left)  p6_type=V-type(Left)  p7_type=V-type(Left)  p8_type=V-type(Left)  p9_type=V-type(Left)  p10_type=V-type(Left)  p11_type=V-type(Left)  p12_type=V-type(Left)  p13_type=V-type(Left)  p14_type=V-type(Left)  p15_type=V-type(Left)  p16_type=V-type(Left)  I_port_shunt_resistance=1e9
  SSN Interface Block (1ph)2 : ssn_lib/SSN Interface Block (1ph)  nb_phase=1  nb_port=2  p1_type=X-type(Left)  p2_type=I-type(Right)  p3_type=X-type(Left)  p4_type=V-type (Right)  p5_type=V-type(Left)  p6_type=V-type(Left)  p7_type=V-type(Left)  p8_type=V-type(Left)  p9_type=V-type(Left)  p10_type=V-type(Left)  p11_type=V-type(Left)  p12_type=V-type(Left)  p13_type=V-type(Left)  p14_type=V-type(Left)  p15_type=V-type(Left)  p16_type=V-type(Left)  I_port_shunt_resistance=1e9
  SSN OLTC xfo v2 : Subsystem  AncestorBlock=artemis/SSN/SSN OLTC/SSN OLTC xfo v2  mask(Norton-Type External Nodal Subsystem){nnode=2, taggg=217x8a73x287908e35664, conntype=2 ports, RLpri=[1e-3 1e-4], Rcore=10000, ensat=off, Lcore=100, Lsat=1, phisat=100, Ts=Ts}
      mask prompts: nnode "Number of Electric nodes"; taggg "Unique Tag Identifier (automatic)"; conntype "Connection type"; RLpri "Primary winding resistance and inductance ([Ohms H])"; Rcore "Core Resistance (Ohms)"; ensat "Enable Saturation"; Lcore "Unsaturated magnetisation inductance (H)"; Lsat "Saturated magnetisation inductance (H)"; phisat "Flux saturation threshold (Weber)"; Ts "Sample Time (s)"
      mask help:
      | Continuously-variable On-Load Tapped Transformer (OLTC) (SSN Custom model)
      |
      | This block implements a 2 winding OLTC saturable transformer in SSN.
      | The model has a variable secondary inductance and resistance as well as turn-ratio.
      | The secondary winding is on the side marked with 'TAP'
      |
      | Mask parameters:
      |    Unique Tag Identifier: unique tag required by SSN to recknonize SSN external models
      |    Primary winding resistance and inductance ([Ohms H])
      |    Core Resistance (Ohms)
      |    Unsaturated magnetisation inductance (H): unsaturated core magnetization inductance
      |    Saturated magnetisation inductance (H): local inductance of the core in the saturated region
      |    Flux saturation threshold (Weber): flux saturation point
      |
      | Signal parameters:
      |
      | Signal inputs:
      |    1st sig: secondary winding resistance (Ohms)
      |    2nd sig: secondary winding inductance (H)
      |    3rd sig: transformer turn ratio k (V_secondary_tapped=k*V_primary)
      |    4th sig:  when set to 1, uses the Backward Euler method for solver. This can be used dynamically during simulation for example to damp numerical oscillations after switching events or after tap changes.
      |
      | Signals ouputs:
      |    1st signal: primary input current (A)
      |    2nd signal: secondary winding current (A)
      |    3rd signal: transformer flux (Wb)
      |
      | Saturation characteristic:
      |          flux
      |             ^              2
      |             |      1       *   <--- slope between point1 and point2 is Lsaturated
      |  phisat  |-----*  <---  this is the knee of flux=f(imag)
      |             |
      |             |
      |             |  <-----slope between origin and point1 is Lunsaturated
      |             *-------------------> imag
      mask init: same as IEEE34bus_2subsystem/SM_34p/Regulator 3/Single Phase SVR_A/Transformer with Taps/SSN OLTC xfo v2
      settings: LibrarySourceBlock=artemis/SSN/SSN OLTC/SSN OLTC xfo v2
      settings: CopyFcn=|
      | str=tempname;
      | str=strrep(str(end-20:end),'_','x');
      | set_param(gcb,'taggg',str);
      | set_param(gcb,'LinkStatus','inactive');
      mask Help: eval('open SSN_OLTC.pdf;');
      mask TypeOptions conntype: 4 ports | 3 ports (primary grounded) | 3 ports (tapped secondary grounded) | 2 ports
      mask Callback conntype:
      | bloc=gcb;
      | conntyp=get_param(bloc,'conntype');
      | nn=fts6_xfo_port_cb(bloc,conntyp);
      | set_param(bloc,'nnode',nn);
      mask Display:
      | plot(a1,a2,a3,a4,b1,b2,b3,b4,c1,c2,c3,c4,c5,c6,c7,c8,c9,c10,c11,c12,c13,c14,c15,c16);
      | color('blue');
      | plot(d1,d2,d3,d4,d5,d6,d7,d8,d9,d10);
  Transfo R2-L2-turnratio : Constant  Value=[0.0001 0.00001 1]
  x : Product  RndMeth=Zero
  L : PMIOPort  Tag=PMCPort  Side=Right
  S : PMIOPort  Port=2  Side=Left
  Isec : Outport
  Vsec : Outport  Port=2
  wires:
  Memory/1 -> Isec/1
  Memory1/1 -> Vsec/1
  " 1"/1 -> Memory/1
  CT1/1 -> " 1"/1
  PT/1 -> "    "/1
  "    "/1 -> Memory1/1
  N/1 -> Fcn/1
  SSN OLTC xfo v2/1(meas) -> "   "/1  "transfo flux (Weber)"
  Back-Euler/1 -> Mux1/2
  Transfo R2-L2-turnratio/1 -> x/2
  x/1 -> Mux1/1
  Mux1/1 -> SSN OLTC xfo v2/1(params)
  Fcn/1 -> x/1
  connections:
  CT1/LConn1 -- L/RConn1
  PT/LConn2 -- Ground1/LConn1
  S/RConn1 -- SSN Interface Block (1ph)/LConn1
  SSN OLTC xfo v2/RConn1 -- SSN Interface Block (1ph)2/LConn1
  SSN OLTC xfo v2/LConn1 -- SSN Interface Block (1ph)/RConn1
  PT/LConn1 -- SSN Interface Block (1ph)2/RConn1 -- CT1/RConn1

== system IEEE34bus_2subsystem/SM_34p/Regulator 4/Single Phase SVR_A/Voltage Regulator Control ==
  Vm : Inport
  Constant : Constant  Value=RegulatorOn
  Tap Changer Control : Subsystem  mask(Tap Changer Control){MinMaxTap=TapMinMax, InitialPosition=InitialTap, MecDelay=TapSelectionTime}
      mask prompts: MinMaxTap "Minimum and maximum tap number [ Min  Max ] :"; InitialPosition "Initial tap position"; MecDelay "Mechanical delay time"
      mask init:
      | if MecDelay<=0,
      | 	MecDelay=1/60;
      | end
  Voltage regulator : Subsystem  mask{Vref=RegulatorVref*120, DeadBand=RegulatorDeadBand*120, TimeDelay=RegulatorDelay}
      mask prompts: Vref "Vref (on 120v base)"; DeadBand "Deadband (on 120v base)"; TimeDelay "Time delay (s)"
  N : Outport
  Tap : Outport  Port=2
  wires:
  Vm/1 -> Voltage regulator/1(Vmes (pu))
  Constant/1 -> Voltage regulator/3(RegOn)
  Tap Changer Control/2(Ready) -> Voltage regulator/2(Ready)
  Voltage regulator/1(Up) -> Tap Changer Control/1("Up ")
  Tap Changer Control/1(TapNo) -> N/1, Tap/1  "Tap"
  Voltage regulator/2(Down) -> Tap Changer Control/2("Down ")

== system IEEE34bus_2subsystem/SM_34p/Regulator 4/Single Phase SVR_B/Line Drop Compensator ==
  note: Vm=Vsec-Isec(Rc+jXc)
  Isec : Inport
  Vsec : Inport  Port=2
  "        " : spsLinearTransformerLib/Linear Transformer  UNITS=SI  NominalPower=[pNom fNom]  winding1=[vNom/ptRatio 1e-7 1e-8]  winding2=[vNom/ptRatio 1e-7 1e-8]  ThreeWindings=off  winding3=[3.15e+005 0.7938 0.084225]  RmLm=[1e5 1e5]  Measurements=None  DataType=on
  "CTS  " : spsControlledCurrentSourceLib/Controlled Current Source  Initialize=on  Source_Type=AC  Amplitude=0  Phase=0  Frequency=0  Measurements=None
  "PTS  " : spsControlledVoltageSourceLib/Controlled Voltage Source  Initialize=on  Source_Type=AC  Amplitude=0  Phase=0  Frequency=0  Measurements=None
  RMS : spsRMSLib/RMS  TrueRMS=on  Freq=60  RMSInit=120  Ts=0
  Raux : spsSeriesRLCBranchLib/Series RLC Branch  LConnTagsString=__new0  RConnTagsString=__new0  BranchType=R  Resistance=1e3  Inductance=1.6 / (120*pi)  SetiL0=off  InitialCurrent=0  Capacitance=1e-6  Setx0=off  InitialVoltage=0  Measurements=None
  Rc+jXc : spsSeriesRLCBranchLib/Series RLC Branch  LConnTagsString=__new0  RConnTagsString=__new0  BranchType=RL  Resistance=Rc  Inductance=Xc / (2*pi*fNom)  SetiL0=off  InitialCurrent=0  Capacitance=1e-6  Setx0=off  InitialVoltage=0  Measurements=None
  VRelay : spsVoltageMeasurementLib/Voltage Measurement  PhasorSimulation=off  OutputType=Complex  PSBequivalent=0
  Vm : Outport
  wires:
  Vsec/1 -> "PTS  "/1
  Isec/1 -> "CTS  "/1
  VRelay/1 -> RMS/1
  RMS/1 -> Vm/1
  connections:
  VRelay/LConn2 -- "PTS  "/LConn1
  "        "/LConn2 -- "CTS  "/LConn1 -- Raux/RConn1 -- Rc+jXc/RConn1
  "CTS  "/RConn1 -- "        "/LConn1 -- Rc+jXc/LConn1 -- Raux/LConn1
  "        "/RConn2 -- VRelay/LConn1
  "PTS  "/RConn1 -- "        "/RConn1

== system IEEE34bus_2subsystem/SM_34p/Regulator 4/Single Phase SVR_B/Transformer with Taps ==
  note: Vsec on Pt Ratio base
  note: Isec on CT Ratio base
  N : Inport
  "   " : Terminator
  "    " : Gain  Gain=1/ptRatio
  " 1" : Gain  Gain=-1/ctRatio
  Back-Euler : Constant
  CT1 : spsCurrentMeasurementLib/Current Measurement  PhasorSimulation=off  OutputType=Complex  PSBequivalent=0
  Fcn : Fcn  Expr=1+0.1*u(1)/16
  Ground1 : spsGroundLib/Ground  LConnTagsString=a
  Memory : Memory
  Memory1 : Memory
  Mux1 : Mux  Inputs=2
  PT : spsVoltageMeasurementLib/Voltage Measurement  PhasorSimulation=off  OutputType=Complex  PSBequivalent=0
  SSN Interface Block (1ph) : ssn_lib/SSN Interface Block (1ph)  nb_phase=1  nb_port=2  p1_type=I-type(Left)  p2_type=X-type(Right)  p3_type=V-type(Left)  p4_type=V-type(Left)  p5_type=V-type(Left)  p6_type=V-type(Left)  p7_type=V-type(Left)  p8_type=V-type(Left)  p9_type=V-type(Left)  p10_type=V-type(Left)  p11_type=V-type(Left)  p12_type=V-type(Left)  p13_type=V-type(Left)  p14_type=V-type(Left)  p15_type=V-type(Left)  p16_type=V-type(Left)  I_port_shunt_resistance=1e9
  SSN Interface Block (1ph)2 : ssn_lib/SSN Interface Block (1ph)  nb_phase=1  nb_port=2  p1_type=X-type(Left)  p2_type=I-type(Right)  p3_type=X-type(Left)  p4_type=V-type (Right)  p5_type=V-type(Left)  p6_type=V-type(Left)  p7_type=V-type(Left)  p8_type=V-type(Left)  p9_type=V-type(Left)  p10_type=V-type(Left)  p11_type=V-type(Left)  p12_type=V-type(Left)  p13_type=V-type(Left)  p14_type=V-type(Left)  p15_type=V-type(Left)  p16_type=V-type(Left)  I_port_shunt_resistance=1e9
  SSN OLTC xfo v2 : Subsystem  AncestorBlock=artemis/SSN/SSN OLTC/SSN OLTC xfo v2  mask(Norton-Type External Nodal Subsystem){nnode=2, taggg=21cxb72ex3f0a0e37a867, conntype=2 ports, RLpri=[1e-3 1e-4], Rcore=10000, ensat=off, Lcore=100, Lsat=1, phisat=100, Ts=Ts}
      mask prompts: nnode "Number of Electric nodes"; taggg "Unique Tag Identifier (automatic)"; conntype "Connection type"; RLpri "Primary winding resistance and inductance ([Ohms H])"; Rcore "Core Resistance (Ohms)"; ensat "Enable Saturation"; Lcore "Unsaturated magnetisation inductance (H)"; Lsat "Saturated magnetisation inductance (H)"; phisat "Flux saturation threshold (Weber)"; Ts "Sample Time (s)"
      mask help:
      | Continuously-variable On-Load Tapped Transformer (OLTC) (SSN Custom model)
      |
      | This block implements a 2 winding OLTC saturable transformer in SSN.
      | The model has a variable secondary inductance and resistance as well as turn-ratio.
      | The secondary winding is on the side marked with 'TAP'
      |
      | Mask parameters:
      |    Unique Tag Identifier: unique tag required by SSN to recknonize SSN external models
      |    Primary winding resistance and inductance ([Ohms H])
      |    Core Resistance (Ohms)
      |    Unsaturated magnetisation inductance (H): unsaturated core magnetization inductance
      |    Saturated magnetisation inductance (H): local inductance of the core in the saturated region
      |    Flux saturation threshold (Weber): flux saturation point
      |
      | Signal parameters:
      |
      | Signal inputs:
      |    1st sig: secondary winding resistance (Ohms)
      |    2nd sig: secondary winding inductance (H)
      |    3rd sig: transformer turn ratio k (V_secondary_tapped=k*V_primary)
      |    4th sig:  when set to 1, uses the Backward Euler method for solver. This can be used dynamically during simulation for example to damp numerical oscillations after switching events or after tap changes.
      |
      | Signals ouputs:
      |    1st signal: primary input current (A)
      |    2nd signal: secondary winding current (A)
      |    3rd signal: transformer flux (Wb)
      |
      | Saturation characteristic:
      |          flux
      |             ^              2
      |             |      1       *   <--- slope between point1 and point2 is Lsaturated
      |  phisat  |-----*  <---  this is the knee of flux=f(imag)
      |             |
      |             |
      |             |  <-----slope between origin and point1 is Lunsaturated
      |             *-------------------> imag
      mask init: same as IEEE34bus_2subsystem/SM_34p/Regulator 3/Single Phase SVR_A/Transformer with Taps/SSN OLTC xfo v2
      settings: LibrarySourceBlock=artemis/SSN/SSN OLTC/SSN OLTC xfo v2
      settings: CopyFcn=|
      | str=tempname;
      | str=strrep(str(end-20:end),'_','x');
      | set_param(gcb,'taggg',str);
      | set_param(gcb,'LinkStatus','inactive');
      mask Help: eval('open SSN_OLTC.pdf;');
      mask TypeOptions conntype: 4 ports | 3 ports (primary grounded) | 3 ports (tapped secondary grounded) | 2 ports
      mask Callback conntype:
      | bloc=gcb;
      | conntyp=get_param(bloc,'conntype');
      | nn=fts6_xfo_port_cb(bloc,conntyp);
      | set_param(bloc,'nnode',nn);
      mask Display:
      | plot(a1,a2,a3,a4,b1,b2,b3,b4,c1,c2,c3,c4,c5,c6,c7,c8,c9,c10,c11,c12,c13,c14,c15,c16);
      | color('blue');
      | plot(d1,d2,d3,d4,d5,d6,d7,d8,d9,d10);
  Transfo R2-L2-turnratio : Constant  Value=[0.0001 0.00001 1]
  x : Product  RndMeth=Zero
  L : PMIOPort  Tag=PMCPort  Side=Right
  S : PMIOPort  Port=2  Side=Left
  Isec : Outport
  Vsec : Outport  Port=2
  wires:
  Fcn/1 -> x/1
  Mux1/1 -> SSN OLTC xfo v2/1(params)
  x/1 -> Mux1/1
  Transfo R2-L2-turnratio/1 -> x/2
  Back-Euler/1 -> Mux1/2
  SSN OLTC xfo v2/1(meas) -> "   "/1  "transfo flux (Weber)"
  N/1 -> Fcn/1
  "    "/1 -> Memory1/1
  PT/1 -> "    "/1
  CT1/1 -> " 1"/1
  " 1"/1 -> Memory/1
  Memory1/1 -> Vsec/1
  Memory/1 -> Isec/1
  connections:
  CT1/RConn1 -- SSN Interface Block (1ph)2/RConn1 -- PT/LConn1
  SSN OLTC xfo v2/LConn1 -- SSN Interface Block (1ph)/RConn1
  SSN OLTC xfo v2/RConn1 -- SSN Interface Block (1ph)2/LConn1
  S/RConn1 -- SSN Interface Block (1ph)/LConn1
  PT/LConn2 -- Ground1/LConn1
  CT1/LConn1 -- L/RConn1

== system IEEE34bus_2subsystem/SM_34p/Regulator 4/Single Phase SVR_B/Voltage Regulator Control ==
  Vm : Inport
  Constant : Constant  Value=RegulatorOn
  Tap Changer Control : Subsystem  mask(Tap Changer Control){MinMaxTap=TapMinMax, InitialPosition=InitialTap, MecDelay=TapSelectionTime}
      mask prompts: MinMaxTap "Minimum and maximum tap number [ Min  Max ] :"; InitialPosition "Initial tap position"; MecDelay "Mechanical delay time"
      mask init:
      | if MecDelay<=0,
      | 	MecDelay=1/60;
      | end
  Voltage regulator : Subsystem  mask{Vref=RegulatorVref*120, DeadBand=RegulatorDeadBand*120, TimeDelay=RegulatorDelay}
      mask prompts: Vref "Vref (on 120v base)"; DeadBand "Deadband (on 120v base)"; TimeDelay "Time delay (s)"
  N : Outport
  Tap : Outport  Port=2
  wires:
  Voltage regulator/2(Down) -> Tap Changer Control/2("Down ")
  Tap Changer Control/1(TapNo) -> Tap/1, N/1  "Tap"
  Voltage regulator/1(Up) -> Tap Changer Control/1("Up ")
  Tap Changer Control/2(Ready) -> Voltage regulator/2(Ready)
  Constant/1 -> Voltage regulator/3(RegOn)
  Vm/1 -> Voltage regulator/1(Vmes (pu))

== system IEEE34bus_2subsystem/SM_34p/Regulator 4/Single Phase SVR_C/Line Drop Compensator ==
  note: Vm=Vsec-Isec(Rc+jXc)
  Isec : Inport
  Vsec : Inport  Port=2
  "        " : spsLinearTransformerLib/Linear Transformer  UNITS=SI  NominalPower=[pNom fNom]  winding1=[vNom/ptRatio 1e-7 1e-8]  winding2=[vNom/ptRatio 1e-7 1e-8]  ThreeWindings=off  winding3=[3.15e+005 0.7938 0.084225]  RmLm=[1e5 1e5]  Measurements=None  DataType=on
  "CTS  " : spsControlledCurrentSourceLib/Controlled Current Source  Initialize=on  Source_Type=AC  Amplitude=0  Phase=0  Frequency=0  Measurements=None
  "PTS  " : spsControlledVoltageSourceLib/Controlled Voltage Source  Initialize=on  Source_Type=AC  Amplitude=0  Phase=0  Frequency=0  Measurements=None
  RMS : spsRMSLib/RMS  TrueRMS=on  Freq=60  RMSInit=120  Ts=0
  Raux : spsSeriesRLCBranchLib/Series RLC Branch  LConnTagsString=__new0  RConnTagsString=__new0  BranchType=R  Resistance=1e3  Inductance=1.6 / (120*pi)  SetiL0=off  InitialCurrent=0  Capacitance=1e-6  Setx0=off  InitialVoltage=0  Measurements=None
  Rc+jXc : spsSeriesRLCBranchLib/Series RLC Branch  LConnTagsString=__new0  RConnTagsString=__new0  BranchType=RL  Resistance=Rc  Inductance=Xc / (2*pi*fNom)  SetiL0=off  InitialCurrent=0  Capacitance=1e-6  Setx0=off  InitialVoltage=0  Measurements=None
  VRelay : spsVoltageMeasurementLib/Voltage Measurement  PhasorSimulation=off  OutputType=Complex  PSBequivalent=0
  Vm : Outport
  wires:
  RMS/1 -> Vm/1
  VRelay/1 -> RMS/1
  Isec/1 -> "CTS  "/1
  Vsec/1 -> "PTS  "/1
  connections:
  "PTS  "/RConn1 -- "        "/RConn1
  "        "/RConn2 -- VRelay/LConn1
  Raux/LConn1 -- Rc+jXc/LConn1 -- "        "/LConn1 -- "CTS  "/RConn1
  Rc+jXc/RConn1 -- Raux/RConn1 -- "CTS  "/LConn1 -- "        "/LConn2
  VRelay/LConn2 -- "PTS  "/LConn1
